simulink model "truck_van_damme"  (R2019a)
settings: Solver=VariableStepAuto  StartTime=0.0  StopTime=100  MaxStep=0.01  RelTol=1e-3
settings Model: EnablePacing=on  Creator=hansae  LastModifiedBy=hansae
settings DebuggingCC: UnconnectedInputMsg=none  UnconnectedOutputMsg=none  UnconnectedLineMsg=none  SFMachineParentedDataDiag=error
settings ModelReferenceCC: EnableRefExpFcnMdlSchedulingChecks=off
settings RTWCC: Description=Generic Real-Time Target

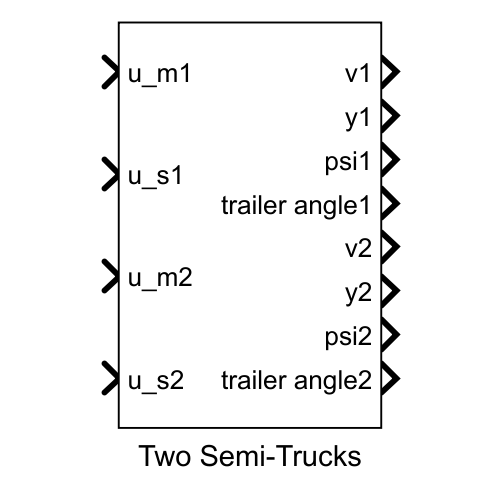
[thumbnail: Simulink's stored preview of the top-level diagram]
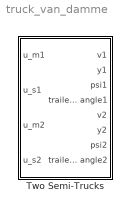
== system truck_van_damme ==
  Two Semi-Trucks : Subsystem

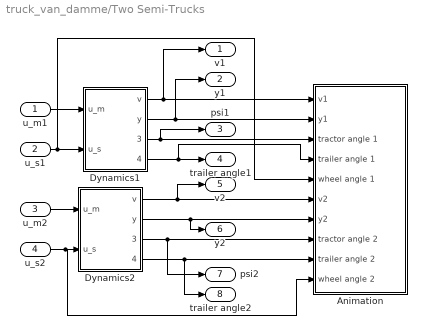
== system truck_van_damme/Two Semi-Trucks ==
  u_m1 : Inport
  u_s1 : Inport  Port=2
  u_m2 : Inport  Port=3
  u_s2 : Inport  Port=4
  Animation : Subsystem
  Dynamics1 : Subsystem  ClipboardFcn=parameters_truck.m
  Dynamics2 : Subsystem  ClipboardFcn=parameters_truck.m
  v1 : Outport
  y1 : Outport  Port=2
  psi1 : Outport  Port=3
  trailer angle1 : Outport  Port=4
  v2 : Outport  Port=5
  y2 : Outport  Port=6
  psi2 : Outport  Port=7
  trailer angle2 : Outport  Port=8
  wires:
  Dynamics1/2(y) -> y1/1, Animation/2(y1)
  u_s1/1 -> Animation/5(wheel angle 1), Dynamics1/2(u_s)
  u_m1/1 -> Dynamics1/1(u_m)
  Dynamics1/3(tractor angle) -> psi1/1, Animation/3(tractor angle 1)
  Dynamics1/4(trailer angle) -> Animation/4(trailer angle 1), trailer angle1/1
  u_s2/1 -> Animation/10(wheel angle 2), Dynamics2/2(u_s)
  Dynamics2/3(tractor angle) -> psi2/1, Animation/8(tractor angle 2)
  Dynamics2/4(trailer angle) -> trailer angle2/1, Animation/9(trailer angle 2)
  Dynamics1/1(v) -> v1/1, Animation/1(v1)
  Dynamics2/1(v) -> v2/1, Animation/6(v2)
  Dynamics2/2(y) -> Animation/7(y2), y2/1
  u_m2/1 -> Dynamics2/1(u_m)

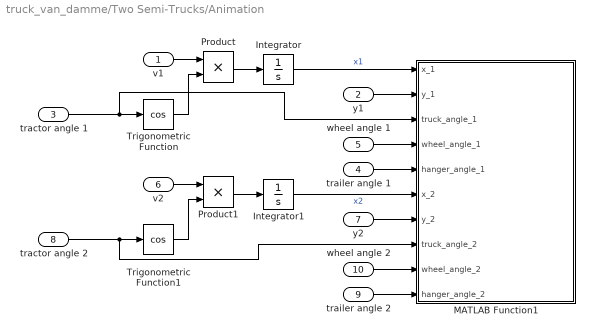
== system truck_van_damme/Two Semi-Trucks/Animation ==
  v1 : Inport
  y1 : Inport  Port=2
  tractor angle 1 : Inport  Port=3
  trailer angle 1 : Inport  Port=4
  wheel angle 1 : Inport  Port=5
  v2 : Inport  Port=6
  y2 : Inport  Port=7
  tractor angle 2 : Inport  Port=8
  trailer angle 2 : Inport  Port=9
  wheel angle 2 : Inport  Port=10
  Integrator : Integrator
  Integrator1 : Integrator
  MATLAB Function1 : MATLAB Function  TreatAsAtomicUnit=on  SystemSampleTime=1/30
  Product : Product
  Product1 : Product
  Trigonometric Function : Trigonometry  Operator=cos
  Trigonometric Function1 : Trigonometry  Operator=cos
  wires:
  Product/1 -> Integrator/1
  Trigonometric Function/1 -> Product/2
  v1/1 -> Product/1
  y1/1 -> MATLAB Function1/2(y_1)
  Integrator/1 -> MATLAB Function1/1(x_1)  "x1"
  tractor angle 1/1 -> MATLAB Function1/3(truck_angle_1), Trigonometric Function/1
  Product1/1 -> Integrator1/1
  Trigonometric Function1/1 -> Product1/2
  v2/1 -> Product1/1
  tractor angle 2/1 -> MATLAB Function1/8(truck_angle_2), Trigonometric Function1/1
  Integrator1/1 -> MATLAB Function1/6(x_2)  "x2"
  y2/1 -> MATLAB Function1/7(y_2)
  trailer angle 1/1 -> MATLAB Function1/5(hanger_angle_1)
  wheel angle 1/1 -> MATLAB Function1/4(wheel_angle_1)
  trailer angle 2/1 -> MATLAB Function1/10(hanger_angle_2)
  wheel angle 2/1 -> MATLAB Function1/9(wheel_angle_2)

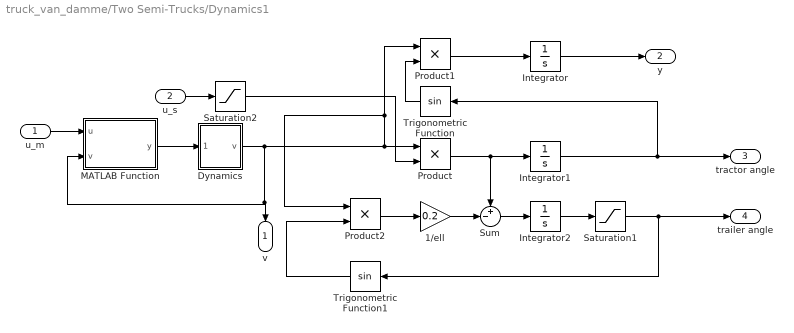
== system truck_van_damme/Two Semi-Trucks/Dynamics1 ==
  u_m : Inport
  u_s : Inport  Port=2
  1/ell : Gain  Gain=0.2
  Dynamics : Subsystem  ClipboardFcn=parameters_truck.m
  Integrator : Integrator  InitialCondition=1.25
  Integrator1 : Integrator
  Integrator2 : Integrator
  MATLAB Function : MATLAB Function  TreatAsAtomicUnit=on
  Product : Product
  Product1 : Product
  Product2 : Product
  Saturation1 : Saturate  UpperLimit=pi/2  LowerLimit=-pi/2
  Saturation2 : Saturate  UpperLimit=pi/4  LowerLimit=-pi/4
  Sum : Sum  Inputs=+-|
  Trigonometric Function : Trigonometry
  Trigonometric Function1 : Trigonometry
  v : Outport
  y : Outport  Port=2
  tractor angle : Outport  Port=3
  trailer angle : Outport  Port=4
  wires:
  Integrator/1 -> y/1
  Product/1 -> Integrator1/1, Sum/1
  Product1/1 -> Integrator/1
  Trigonometric Function/1 -> Product1/2
  Integrator2/1 -> Saturation1/1
  Trigonometric Function1/1 -> Product2/2
  Product2/1 -> 1/ell/1
  Sum/1 -> Integrator2/1
  1/ell/1 -> Sum/2
  Saturation2/1 -> Product/2
  Integrator1/1 -> tractor angle/1, Trigonometric Function/1
  Saturation1/1 -> trailer angle/1, Trigonometric Function1/1
  u_s/1 -> Saturation2/1
  MATLAB Function/1(y) -> Dynamics/1(u_m)
  u_m/1 -> MATLAB Function/1(u)
  Dynamics/1(v) -> v/1, MATLAB Function/2(v), Product2/1, Product1/1, Product/1

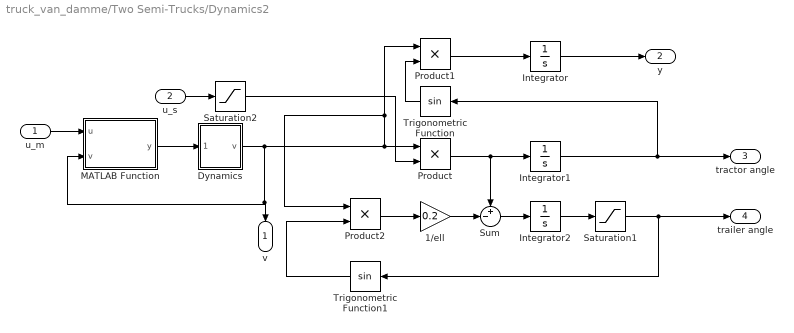
== system truck_van_damme/Two Semi-Trucks/Dynamics2 ==
  u_m : Inport
  u_s : Inport  Port=2
  1/ell : Gain  Gain=0.2
  Dynamics : Subsystem  ClipboardFcn=parameters_truck.m
  Integrator : Integrator  InitialCondition=-1.25
  Integrator1 : Integrator
  Integrator2 : Integrator
  MATLAB Function : MATLAB Function  TreatAsAtomicUnit=on
  Product : Product
  Product1 : Product
  Product2 : Product
  Saturation1 : Saturate  UpperLimit=pi/2  LowerLimit=-pi/2
  Saturation2 : Saturate  UpperLimit=pi/4  LowerLimit=-pi/4
  Sum : Sum  Inputs=+-|
  Trigonometric Function : Trigonometry
  Trigonometric Function1 : Trigonometry
  v : Outport
  y : Outport  Port=2
  tractor angle : Outport  Port=3
  trailer angle : Outport  Port=4
  wires:
  Integrator/1 -> y/1
  Product/1 -> Integrator1/1, Sum/1
  Product1/1 -> Integrator/1
  Trigonometric Function/1 -> Product1/2
  Integrator2/1 -> Saturation1/1
  Trigonometric Function1/1 -> Product2/2
  Product2/1 -> 1/ell/1
  Sum/1 -> Integrator2/1
  1/ell/1 -> Sum/2
  Saturation2/1 -> Product/2
  Integrator1/1 -> tractor angle/1, Trigonometric Function/1
  Saturation1/1 -> trailer angle/1, Trigonometric Function1/1
  u_s/1 -> Saturation2/1
  MATLAB Function/1(y) -> Dynamics/1(u_m)
  u_m/1 -> MATLAB Function/1(u)
  Dynamics/1(v) -> v/1, MATLAB Function/2(v), Product2/1, Product1/1, Product/1

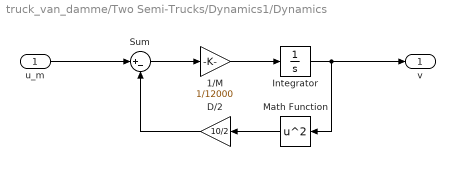
== system truck_van_damme/Two Semi-Trucks/Dynamics1/Dynamics ==
  u_m : Inport
  1/M : Gain  Gain=1/12000
  D/2 : Gain  Gain=10/2
  Integrator : Integrator
  Math Function : Math  Operator=square  SaturateOnIntegerOverflow=on
  Sum : Sum  Inputs=|+-
  v : Outport
  wires:
  Integrator/1 -> v/1, Math Function/1
  Sum/1 -> 1/M/1
  u_m/1 -> Sum/1
  1/M/1 -> Integrator/1
  D/2/1 -> Sum/2
  Math Function/1 -> D/2/1

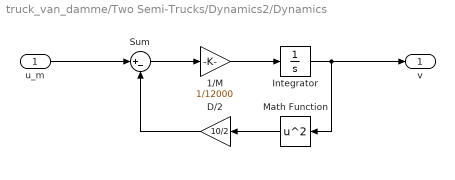
== system truck_van_damme/Two Semi-Trucks/Dynamics2/Dynamics ==
  u_m : Inport
  1/M : Gain  Gain=1/12000
  D/2 : Gain  Gain=10/2
  Integrator : Integrator
  Math Function : Math  Operator=square  SaturateOnIntegerOverflow=on
  Sum : Sum  Inputs=|+-
  v : Outport
  wires:
  Integrator/1 -> v/1, Math Function/1
  Sum/1 -> 1/M/1
  u_m/1 -> Sum/1
  1/M/1 -> Integrator/1
  D/2/1 -> Sum/2
  Math Function/1 -> D/2/1

== matlab function truck_van_damme/Two Semi-Trucks/Dynamics1/MATLAB Function ==
  data: u input; y output; v input
function y = saturation(u,v)
    Pmax = 400000;
    epsilon = 0.1;
    
    sat = Pmax/sqrt(v^2+epsilon);
    y = max(min(u,sat),-sat);

== matlab function truck_van_damme/Two Semi-Trucks/Dynamics2/MATLAB Function ==
  data: u input; y output; v input
function y = saturation(u,v)
    Pmax = 400000;
    epsilon = 0.1;
    
    sat = Pmax/sqrt(v^2+epsilon);
    y = max(min(u,sat),-sat);

== matlab function truck_van_damme/Two Semi-Trucks/Animation/MATLAB Function1 ==
  settings: updateMethod=DISCRETE
  data: x_1 input; y_1 input; truck_angle_1 input; wheel_angle_1 input; hanger_angle_1 input; x_2 input; y_2 input; truck_angle_2 input; wheel_angle_2 input; hanger_angle_2 input
function plot_truck( ...
    x_1,y_1,truck_angle_1,wheel_angle_1,hanger_angle_1, ...
    x_2,y_2,truck_angle_2,wheel_angle_2,hanger_angle_2)

    % Parameters
    l = 8;
    persistent Truck_1 Truck_2;

    % Plotting Truck
    if isempty(Truck_1)
        [Truck_1, Truck_2] = initialize_plot();
    else
        update_truck_position(Truck_1,Truck_2, ...
            x_1,y_1,truck_angle_1,wheel_angle_1,hanger_angle_1, ...
            x_2,y_2,truck_angle_2,wheel_angle_2,hanger_angle_2);
    end    

    drawnow;

    % Functions
    function [Truck_1, Truck_2] = initialize_plot()
        % Create figure
        figure('position',[100,100,1500,500]);
        clf; grid on; hold on; daspect([1,1,1]);
        xlim([-20, 50])
        ylim([-10, 10])
    
        % Road
        plot([-5000,5000],[-4,-4],'k','linewidth',3);
        plot([-5000,5000],[4,4],'k','linewidth',3);
        plot([-5000,5000],[0,0],'y','linewidth',3);

        % Truck 1
        Truck_1               = hgtransform('parent',gca);
        Left_front_wheel_1    = hgtransform('parent',Truck_1);
        Right_front_wheel_1   = hgtransform('parent',Truck_1);
        Hanger_1              = hgtransform('parent',Truck_1);

        % Back front wheels
        rectangle('Position',[l/2,-l/100,l/8,l/40],'parent',Truck_1,'edgecolor','k','linewidth',2,'FaceColor','w')
        rectangle('Position',[l/2,l-2*l/3-(l/40-l/100),l/8,l/40],'parent',Truck_1,'edgecolor','k','linewidth',2,'FaceColor','w')
        % Front front wheel
        rectangle('Position',[2*l/3+l/20,-l/100,l/8,l/40],'parent',Right_front_wheel_1,'edgecolor','k','linewidth',2,'FaceColor','w')
        rectangle('Position',[2*l/3+l/20,l-2*l/3-(l/40-l/100),l/8,l/40],'parent',Left_front_wheel_1,'edgecolor','k','linewidth',2,'FaceColor','w')
        % Front
        rectangle('Position',[2*l/3+l/32,0,l-2*l/3-l/32,l-2*l/3],'parent',Truck_1,'edgecolor','k','linewidth',2,'FaceColor','w')
        rectangle('Position',[l/2,3*l/8-l/3,2*l/3-11*l/18+(11*l/18-l/2)+l/32,l-3*l/4],'parent',Truck_1,'edgecolor','k','linewidth',2,'FaceColor','w')
        % Window
        rectangle('Position',[7*l/8,0,l/8,l-2*l/3],'parent',Truck_1,'edgecolor','k','linewidth',2,'FaceColor','w')
        
        % Back wheels
        rectangle('Position',[-l/2+l/8,-l/100,l/8,l/40],'parent',Hanger_1,'edgecolor','k','linewidth',2,'FaceColor','w')
        rectangle('Position',[-l/2+l/8,l-2*l/3-(l/40-l/100),l/8,l/40],'parent',Hanger_1,'edgecolor','k','linewidth',2,'FaceColor','w')
        % Hanger
        rectangle('Position',[-l/2,0,11*l/18+l/2,l-2*l/3],'parent',Hanger_1,'edgecolor','k','linewidth',2,'FaceColor','w')

        children = get(Truck_1, 'Children');
        reorderedChildren = [children(6); children(1:5); children(7:8)];
        set(Truck_1, 'Children', reorderedChildren);

        % Truck 2
        Truck_2               = hgtransform('parent',gca);
        Left_front_wheel_2    = hgtransform('parent',Truck_2);
        Right_front_wheel_2   = hgtransform('parent',Truck_2);
        Hanger_2              = hgtransform('parent',Truck_2);

        % Back front wheels
        rectangle('Position',[l/2,-l/100,l/8,l/40],'parent',Truck_2,'edgecolor','k','linewidth',2,'FaceColor','w')
        rectangle('Position',[l/2,l-2*l/3-(l/40-l/100),l/8,l/40],'parent',Truck_2,'edgecolor','k','linewidth',2,'FaceColor','w')
        % Front front wheel
        rectangle('Position',[2*l/3+l/20,-l/100,l/8,l/40],'parent',Right_front_wheel_2,'edgecolor','k','linewidth',2,'FaceColor','w')
        rectangle('Position',[2*l/3+l/20,l-2*l/3-(l/40-l/100),l/8,l/40],'parent',Left_front_wheel_2,'edgecolor','k','linewidth',2,'FaceColor','w')
        % Front
        rectangle('Position',[2*l/3+l/32,0,l-2*l/3-l/32,l-2*l/3],'parent',Truck_2,'edgecolor','k','linewidth',2,'FaceColor','w')
        rectangle('Position',[l/2,3*l/8-l/3,2*l/3-11*l/18+(11*l/18-l/2)+l/32,l-3*l/4],'parent',Truck_2,'edgecolor','k','linewidth',2,'FaceColor','w')
        % Window
        rectangle('Position',[7*l/8,0,l/8,l-2*l/3],'parent',Truck_2,'edgecolor','k','linewidth',2,'FaceColor','w')
        
        % Back wheels
        rectangle('Position',[-l/2+l/8,-l/100,l/8,l/40],'parent',Hanger_2,'edgecolor','k','linewidth',2,'FaceColor','w')
        rectangle('Position',[-l/2+l/8,l-2*l/3-(l/40-l/100),l/8,l/40],'parent',Hanger_2,'edgecolor','k','linewidth',2,'FaceColor','w')
        % Hanger
        rectangle('Position',[-l/2,0,11*l/18+l/2,l-2*l/3],'parent',Hanger_2,'edgecolor','k','linewidth',2,'FaceColor','w')

        children = get(Truck_2, 'Children');
        reorderedChildren = [children(6); children(1:5); children(7:8)];
        set(Truck_2, 'Children', reorderedChildren);

    end
    
    function update_truck_position(Truck_1,Truck_2, ...
            x_1,y_1,truck_angle_1,wheel_angle_1,hanger_angle_1, ...
            x_2,y_2,truck_angle_2,wheel_angle_2,hanger_angle_2)
        if ishandle(Truck_1)
            
            % Truck 1
            set(Truck_1, 'Matrix', makehgtform('translate', [x_1, y_1, 0], 'zrotate', truck_angle_1, 'translate', [-l/6-l/16-l/4-l/12, -l/2+l/3, 0]));
            
            children = get(Truck_1, 'Children');
            set(children(8), 'Matrix', makehgtform('translate', -[-(2*l/3+l/20)-l/16, -(l-2*l/3-(l/40-l/100))-l/80, 0], 'zrotate', -wheel_angle_1, 'translate', [-(2*l/3+l/20)-l/16, -(l-2*l/3-(l/40-l/100))-l/80, 0]));
            set(children(7), 'Matrix', makehgtform('translate', -[-(2*l/3+l/20)-l/16, l/100-l/80, 0], 'zrotate', -wheel_angle_1, 'translate', [-(2*l/3+l/20)-l/16, l/100-l/80, 0]));

            set(children(1), 'Matrix', makehgtform('translate', -[-l/6-l/16-l/4-l/12, -l/2+l/3, 0],'zrotate', -hanger_angle_1,'translate', [-l/6-l/16-l/4-l/12, -l/2+l/3, 0]));
    
            % Truck 2
            set(Truck_2, 'Matrix', makehgtform('translate', [x_2, y_2, 0], 'zrotate', truck_angle_2, 'translate', [-l/6-l/16-l/4-l/12, -l/2+l/3, 0]));
            
            children = get(Truck_2, 'Children');
            set(children(8), 'Matrix', makehgtform('translate', -[-(2*l/3+l/20)-l/16, -(l-2*l/3-(l/40-l/100))-l/80, 0], 'zrotate', -wheel_angle_2, 'translate', [-(2*l/3+l/20)-l/16, -(l-2*l/3-(l/40-l/100))-l/80, 0]));
            set(children(7), 'Matrix', makehgtform('translate', -[-(2*l/3+l/20)-l/16, l/100-l/80, 0], 'zrotate', -wheel_angle_2, 'translate', [-(2*l/3+l/20)-l/16, l/100-l/80, 0]));

            set(children(1), 'Matrix', makehgtform('translate', -[-l/6-l/16-l/4-l/12, -l/2+l/3, 0],'zrotate', -hanger_angle_2,'translate', [-l/6-l/16-l/4-l/12, -l/2+l/3, 0]));
    
            xlim([-20, 50] + x_1)
            ylim([-10, 10] + y_1)
        end
    end
end
